simulink model "HIGHslx"  (R2020a)
settings: Solver=VariableStepAuto  StartTime=0.0  StopTime=10.0  RelTol=1e-3
libraries: fuzblock x1
settings Model: Creator=macbookpro  LastModifiedBy=Mayaar Alaa
settings DataIOCC: ReturnWorkspaceOutputs=off
settings DebuggingCC: ArithmeticOperatorsInVariantConditions=warning
settings SFSimCC: SimUseLocalCustomCode=off  CustomCodeUndefinedFunction=UseInterfaceOnly
settings RTWCC: RTWUseLocalCustomCode=off

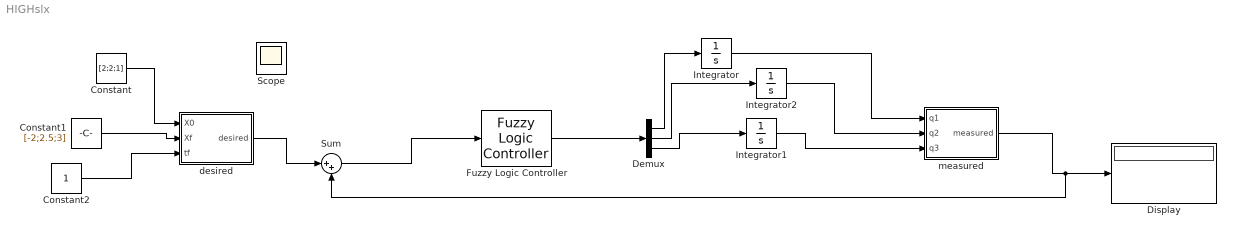
== system HIGHslx ==
  Constant : Constant  Value=[2;2;1]
  Constant1 : Constant  Value=[-2;2.5;3]
  Constant2 : Constant
  Demux : Demux  Outputs=3
  Display : Display
  Fuzzy Logic Controller : fuzblock/Fuzzy Logic  Controller  FIS='fuzzyy.fis'  OutputSampleNumber=101  DataType=double  FuzzifiedInputs=off  RuleFiringStrengths=off  RuleOutputs=off  AggregatedOutputs=off  SimulateUsing=Interpreted execution  OutOfRangeInputValueMessage=warning  NoRuleFiredMessage=warning  EmptyOutputFuzzySetMessage=warning
  Integrator : Integrator
  Integrator1 : Integrator
  Integrator2 : Integrator
  Sum : Sum  Inputs=|++
  desired : MATLAB Function  TreatAsAtomicUnit=on
  measured : MATLAB Function  TreatAsAtomicUnit=on
  Scope : Scope
  wires:
  Constant/1 -> desired/1(X0)
  Constant1/1 -> desired/2(Xf)
  Constant2/1 -> desired/3(tf)
  measured/1(measured) -> Sum/2, Display/1
  desired/1(desired) -> Sum/1
  Demux/2 -> Integrator2/1
  Demux/1 -> Integrator/1
  Integrator/1 -> measured/1(q1)
  Sum/1 -> Fuzzy Logic Controller/1
  Fuzzy Logic Controller/1 -> Demux/1
  Demux/3 -> Integrator1/1
  Integrator2/1 -> measured/2(q2)
  Integrator1/1 -> measured/3(q3)

== matlab function HIGHslx/measured ==
  data: q1 input; measured output; q2 input; q3 input
function measured = m(q1,q2,q3)
theta = 0 ; d = 5 ; a=0 ; alpha = 0 
T01 = [cosd(theta)  -sind(theta)*cosd(alpha) sind(theta)*sind(alpha) a*cosd(theta) ;
       sind(theta) cosd(theta)*cosd(alpha) -cosd(theta)*sind(alpha) a*sind(theta);
       0 sind(alpha) cosd(alpha) d;
       0 0 0 1]
   theta = q1 ; d = 0 ; a=5 ; alpha = 90 ; 
   T12 = [cosd(theta)  -sind(theta)*cosd(alpha) sind(theta)*sind(alpha) a*cosd(theta) ;
       sind(theta) cosd(theta)*cosd(alpha) -cosd(theta)*sind(alpha) a*sind(theta);
       0 sind(alpha) cosd(alpha) d;
       0 0 0 1]
   theta = q2 ; d = 0 ; a=5 ; alpha = 0 ;
   T23 = [cosd(theta)  -sind(theta)*cosd(alpha) sind(theta)*sind(alpha) a*cosd(theta) ;
       sind(theta) cosd(theta)*cosd(alpha) -cosd(theta)*sind(alpha) a*sind(theta);
       0 sind(alpha) cosd(alpha) d;
       0 0 0 1]
   theta = q3 ; d = 10 ; a=0 ; alpha = 0 ;
   T67 = [cosd(theta)  -sind(theta)*cosd(alpha) sind(theta)*sind(alpha) a*cosd(theta) ;
       sind(theta) cosd(theta)*cosd(alpha) -cosd(theta)*sind(alpha) a*sind(theta);
       0 sind(alpha) cosd(alpha) d;
       0 0 0 1]
  
     x = T01*T12*T23*T67 
       
      measured = [ x(1,4) ; x(2,4) ; x(3,4) ]
end

== matlab function HIGHslx/desired ==
  data: X0 input; desired output; Xf input; tf input
function desired = task_traj_3(X0, Xf, tf)

% linear
x0= X0(1);
y0= X0(2);
z0= X0(3);
xf= Xf(1);
yf= Xf(2);
zf= Xf(3);

alphax= (xf-x0)/tf
alphay= (yf-y0)/tf
alphaz= (zf-z0)/tf
t=0
   xt= x0+(alphax*t);
    yt= y0+(alphay*t);
    zt= z0+(alphaz*t);
X= [ xt ; yt  ; zt ] 

 
for i = 0.0:0.1:tf
    
    
    t = i 
    xt= x0+(alphax*t);
    yt= y0+(alphay*t);
    zt= z0+(alphaz*t);
      X= [ xt ; yt  ; zt ] 
   q_0=[232.0379;193.3135;60.0000]
      X = [X(1) ; X(2); X(3)]
      q_i=[q_0(1);q_0(2); q_0(3)];
      q1 = q_i(1);
      q2 = q_i(2);
      q3 = q_i(3);
      
      
       H = [ (pi*cos((pi*q1)/180))/18 - (pi*sin((pi*q1)/180))/36 - (pi*cos((pi*q2)/180)*sin((pi*q1)/180))/36, -(pi*cos((pi*q1)/180)*sin((pi*q2)/180))/36, 0 ;
           (pi*cos((pi*q1)/180))/36 + (pi*sin((pi*q1)/180))/18 + (pi*cos((pi*q1)/180)*cos((pi*q2)/180))/36, -(pi*sin((pi*q1)/180)*sin((pi*q2)/180))/36, 0;
                                                                                                       0,                   (pi*cos((pi*q2)/180))/36, 0]
 
%      
%     L = [ 5*cos((pi*q1)/180) + 5*cos((pi*q1)/180)*cos((pi*q2)/180) + 10*sin((pi*q5)/180)*(sin((pi*q1)/180)*sin((pi*q4)/180) + cos((pi*q1)/180)*cos((pi*q2)/180)*cos((pi*q3)/180)*cos((pi*q4)/180) - cos((pi*q1)/180)*cos((pi*q4)/180)*sin((pi*q2)/180)*sin((pi*q3)/180)) + 10*sin((pi*(q2 + q3))/180)*cos((pi*q1)/180)*cos((pi*q5)/180) + 10*cos((pi*q1)/180)*cos((pi*q2)/180)*sin((pi*q3)/180) + 10*cos((pi*q1)/180)*cos((pi*q3)/180)*sin((pi*q2)/180);
%                   5*sin((pi*q1)/180) + 5*cos((pi*q2)/180)*sin((pi*q1)/180) - 10*sin((pi*q5)/180)*(cos((pi*q1)/180)*sin((pi*q4)/180) - cos((pi*q2)/180)*cos((pi*q3)/180)*cos((pi*q4)/180)*sin((pi*q1)/180) + cos((pi*q4)/180)*sin((pi*q1)/180)*sin((pi*q2)/180)*sin((pi*q3)/180)) + 10*cos((pi*q2)/180)*sin((pi*q1)/180)*sin((pi*q3)/180) + 10*cos((pi*q3)/180)*sin((pi*q1)/180)*sin((pi*q2)/180) + 10*sin((pi*(q2 + q3))/180)*cos((pi*q5)/180)*sin((pi*q1)/180);
%                   5*sin((pi*q2)/180) - 10*cos((pi*(q2 + q3))/180) + 5*sin((pi*(q2 + q3))/180)*sin((pi*(q4 + q5))/180) - 10*cos((pi*(q2 + q3))/180)*cos((pi*q5)/180) - 5*sin((pi*(q2 + q3))/180)*sin((pi*(q4 - q5))/180) + 5 ]                                                                                                                                                                  
%   
%               
    ql= pinv(H)*X;
     q_i = q_i - ql ;
      
      
   for   i = 0 : 3
     
  
   
  
     q1 = q_i(1);
      q2 = q_i(2);
      q3 = q_i(3);
      
      
     H = [ (pi*cos((pi*q1)/180))/18 - (pi*sin((pi*q1)/180))/36 - (pi*cos((pi*q2)/180)*sin((pi*q1)/180))/36, -(pi*cos((pi*q1)/180)*sin((pi*q2)/180))/36, 0 ;
           (pi*cos((pi*q1)/180))/36 + (pi*sin((pi*q1)/180))/18 + (pi*cos((pi*q1)/180)*cos((pi*q2)/180))/36, -(pi*sin((pi*q1)/180)*sin((pi*q2)/180))/36, 0;
                                                                                                       0,                   (pi*cos((pi*q2)/180))/36, 0]
 
%     L = [ 5*cos((pi*q1)/180) + 5*cos((pi*q1)/180)*cos((pi*q2)/180) + 10*sin((pi*q5)/180)*(sin((pi*q1)/180)*sin((pi*q4)/180) + cos((pi*q1)/180)*cos((pi*q2)/180)*cos((pi*q3)/180)*cos((pi*q4)/180) - cos((pi*q1)/180)*cos((pi*q4)/180)*sin((pi*q2)/180)*sin((pi*q3)/180)) + 10*sin((pi*(q2 + q3))/180)*cos((pi*q1)/180)*cos((pi*q5)/180) + 10*cos((pi*q1)/180)*cos((pi*q2)/180)*sin((pi*q3)/180) + 10*cos((pi*q1)/180)*cos((pi*q3)/180)*sin((pi*q2)/180);
%                   5*sin((pi*q1)/180) + 5*cos((pi*q2)/180)*sin((pi*q1)/180) - 10*sin((pi*q5)/180)*(cos((pi*q1)/180)*sin((pi*q4)/180) - cos((pi*q2)/180)*cos((pi*q3)/180)*cos((pi*q4)/180)*sin((pi*q1)/180) + cos((pi*q4)/180)*sin((pi*q1)/180)*sin((pi*q2)/180)*sin((pi*q3)/180)) + 10*cos((pi*q2)/180)*sin((pi*q1)/180)*sin((pi*q3)/180) + 10*cos((pi*q3)/180)*sin((pi*q1)/180)*sin((pi*q2)/180) + 10*sin((pi*(q2 + q3))/180)*cos((pi*q5)/180)*sin((pi*q1)/180);
%                   5*sin((pi*q2)/180) - 10*cos((pi*(q2 + q3))/180) + 5*sin((pi*(q2 + q3))/180)*sin((pi*(q4 + q5))/180) - 10*cos((pi*(q2 + q3))/180)*cos((pi*q5)/180) - 5*sin((pi*(q2 + q3))/180)*sin((pi*(q4 - q5))/180) + 5 ] ;                                                                                                                                                                 

              
    ql= pinv(H)*X ;
     q_i = q_i - ql ;
       
               
   end
     
           q3 = q_i

  
   
  
    
    
end
desired = [xt;yt;zt]

  end
